simulink model "mainSimulink_localPi"  (R2021a)
settings: Solver=VariableStepAuto  StartTime=0.0  StopTime=inf  FixedStep=samplingTime  RelTol=1e-3
model workspace (MATLAB code in the model file):
  | %% Simulink settings
  | controllerFile = 'directFFcontroller';
  | set_param('mainSimulink_localPi/Subsystem Reference', 'ReferencedSubsystem', controllerFile);
  | %% Display settings
  | scopeTimeSpan = 30;
  | 
  | %% Robot settings (must match Python)
  | sensorFreq = 250;
  | actuatorFreq = 250;
  | PiAddress = '192.168.4.1';
  | PiTCPport = 12345;
  | dataSize = 3;
  | actuatorMin = [0,0,0];                                  %Min relative pressure for actuators [kPa per actuator]
  | actuatorMax = [20,20,20];                                 %Max relative pressure for actuators [kPa per actuator]
  | regulatorMin = -100;                                %Min relative pressure output for regulators [kPa, same for all regulators]
  | regulatorMax = 100;                                 %Max relative pressure output for regulators [kPa, same for all regulators]
  | sensorSamplingTime = 1/sensorFreq;
  | actuatorTime = 1/actuatorFreq;
  | 
  | %% Unity communication settings (must match Unity)
  | UnityAddress = '127.0.0.1';                         %address for Matlab-Unity communication. 127.0.0.1 means local
  | UnityTCPport = 26950;                               %make sure that this port matches the one chosen in Unity
  | nrMessages = 3;                                     %nr of values that you are reading per packet. Depends on your Unity settings
  | UnitysampleFrequency = 120;                         %frequency on Simulink checking TCP connection
  | 
  | %%%ONLY EDIT WHEN THE UNITY MESSAGE TYPE OR HEADER CHANGES%%
  | headerWidth = 12;                                   %nr of bytes in message header (before actual message)
  | signalWidth = 8;                                    %length of each value in message, depends on data type (which is double for now, which is 8 bytes)
  | messageWidth = nrMessages .* signalWidth;           %length of message without header
  | totalMessageWidth = headerWidth + messageWidth;     %length of total packet
  | UnitySamplingTime = 1/UnitysampleFrequency;
undefined symbols (not defined in the file): f
libraries: slrealtimeutilitieslib x4, etargetslib x4, slrealtimeiplib x3, instrumentlib x2
settings Model: EnablePacing=on  Creator=chukh  LastModifiedBy=20210123

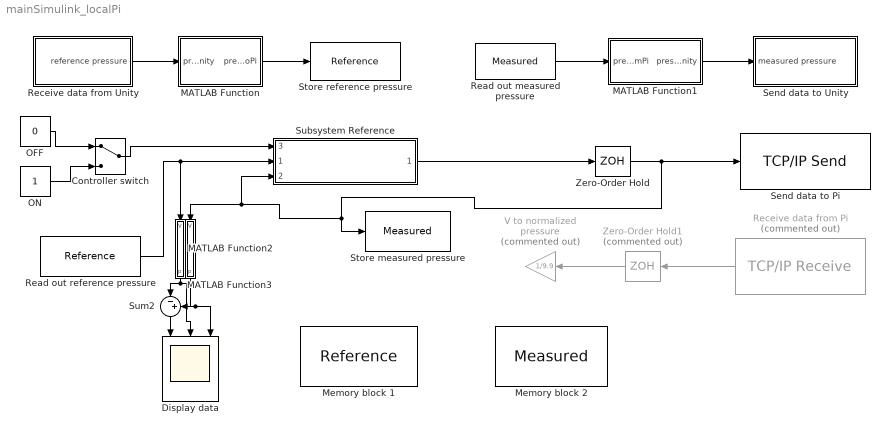
== system mainSimulink_localPi ==
  Controller switch : ManualSwitch
  Display data : Scope  NumInputPorts=3
  MATLAB Function : MATLAB Function  TreatAsAtomicUnit=on
  MATLAB Function1 : MATLAB Function  TreatAsAtomicUnit=on
  MATLAB Function2 : MATLAB Function  TreatAsAtomicUnit=on
  MATLAB Function3 : MATLAB Function  TreatAsAtomicUnit=on
  Memory block 1 : DataStoreMemory  DataStoreName=Reference  ReadBeforeWriteMsg=warning  WriteAfterWriteMsg=warning  WriteAfterReadMsg=warning  InitialValue=zeros(1,dataSize)  ShowAdditionalParam=off  Dimensions=[1 dataSize]
  Memory block 2 : DataStoreMemory  DataStoreName=Measured  ReadBeforeWriteMsg=warning  WriteAfterWriteMsg=warning  WriteAfterReadMsg=warning  InitialValue=zeros(1,dataSize)  ShowAdditionalParam=off  Dimensions=[1 dataSize]
  OFF : Constant  Value=0
  ON : Constant
  Read out measured pressure : DataStoreRead  DataStoreName=Measured  IndexOptions=Index vector (dialog)  Indices=1  OutputSizes=1
  Read out reference pressure : DataStoreRead  DataStoreName=Reference  IndexOptions=Index vector (dialog)  Indices=1  OutputSizes=1
  Receive data from Pi : instrumentlib/TCP//IP Receive  Commented=on  Host=192.168.4.1  Port=PiTCPport  DataSize=dataSize  EnableBlockingMode=on  Timeout=0.5  SampleTime=sensorSamplingTime  DataType=double  ByteOrder=LittleEndian  ASCIIFormatting=%f,  Terminator=LF
  Receive data from Unity : Subsystem
  Send data to Pi : instrumentlib/TCP//IP Send  Host=192.168.4.1  Port=PiTCPport  EnableBlockingMode=on  Timeout=0.5  ByteOrder=LittleEndian  TransferDelay=on
  Send data to Unity : Subsystem
  Store measured pressure : DataStoreWrite  DataStoreName=Measured  IndexOptions=Index vector (dialog)  Indices=1  OutputSizes=1
  Store reference pressure : DataStoreWrite  DataStoreName=Reference  IndexOptions=Index vector (dialog)  Indices=1  OutputSizes=1
  Subsystem Reference : Subsystem  ReferencedSubsystem=directFFcontroller
      settings: PortSchema="{\"entries\":[{\"content\":{\"sides\":[{\"content\":{\"connectorIds\":[\"In3\",\"In1\",\"In2\"]},\"type\":\"ConnectorPlacement.EquallySpacedRectSide\",\"uuid\":\"e7b3a722-e0eb-4523-936c-9c3b79c2c41f\"},{\"content\":{\"connectorIds\":[\"Out1\"],\"side\":\"RIGHT\"},\"type\":\"ConnectorPlacement.EquallySpacedRectSide\",\"uuid\":\"1532b6ae-993f-4a88-9279-fc9a4eded03a\"},{\"content\":{\"connectorIds\":[],\"side\":\"TOP\"},\"type\":\"ConnectorPlacement.EquallySpacedRectSide\",\"uuid\":\"9848284d-3c0a-4259-bac0-7c6aae442a0e\"}]},\"type\":\"ConnectorPlacement.EquallySpacedConnector\",\"uuid\":\"d62a861a-c088-4a48-af1e-4b6a4475476a\"}],\"packageUris\":[\"http://schema.mathworks.com/mf0/Connector/R2020b\"],\"version\":\"1.0\"}"
  Sum2 : Sum  Inputs=|-+
  V to normalized pressure : Gain  Commented=on  Gain=1/9.9
  Zero-Order Hold : ZeroOrderHold  SampleTime=actuatorTime
  Zero-Order Hold1 : ZeroOrderHold  Commented=on  SampleTime=actuatorTime
  wires:
  Zero-Order Hold1/1 -> V to normalized pressure/1
  MATLAB Function2/1(p) -> Sum2/1, Display data/2
  MATLAB Function3/1(p) -> Sum2/2, Display data/3
  Read out reference pressure/1 -> MATLAB Function2/1(V), Subsystem Reference/1
  Sum2/1 -> Display data/1
  Receive data from Unity/1("reference pressure ") -> MATLAB Function/1(pressureFromUnity)
  MATLAB Function/1(pressureToPi) -> Store reference pressure/1
  Read out measured pressure/1 -> MATLAB Function1/1(pressureFromPi)
  Receive data from Pi/1 -> Zero-Order Hold1/1
  Zero-Order Hold/1 -> Subsystem Reference/2, MATLAB Function3/1(V), Store measured pressure/1, Send data to Pi/1
  Subsystem Reference/1 -> Zero-Order Hold/1
  MATLAB Function1/1(pressureToUnity) -> Send data to Unity/1(measured pressure)
  OFF/1 -> Controller switch/1
  ON/1 -> Controller switch/2
  Controller switch/1 -> Subsystem Reference/3

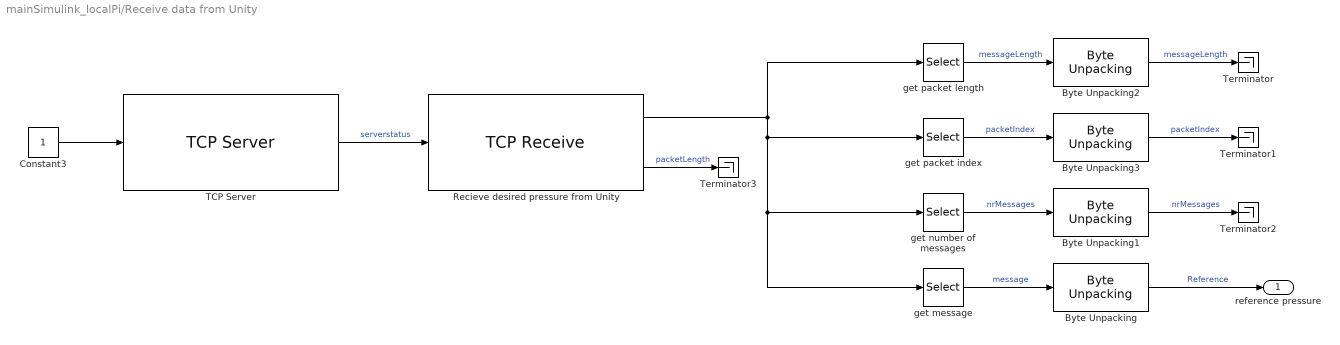
== system mainSimulink_localPi/Receive data from Unity ==
  Byte Unpacking{,1..3} (4 alike) : slrealtimeutilitieslib/Byte Unpacking
      settings: SourceProductBaseCode=XP
  Constant3 : Constant  OutDataTypeStr=double
  Recieve desired pressure from Unity : slrealtimeiplib/TCP Receive  Priority=1  socketAddPortVal=Server: UnityAddress:UnityTCPport  rcvWidth=totalMessageWidth  sampleTime=UnitySamplingTime
      settings: SourceProductBaseCode=XP
  TCP Server : slrealtimeiplib/TCP Server  Priority=-1  useHostTargetConn=off  serverAddress=UnityAddress  serverPort=UnityTCPport
      settings: SourceProductBaseCode=XP
  Terminator{,1..3} (4 alike) : Terminator
  get message : Selector  InputPortWidth=totalMessageWidth  IndexOptions=Index vector (dialog)  Indices=[headerWidth+1:totalMessageWidth]  OutputSizes=1
  get number of messages : Selector  InputPortWidth=totalMessageWidth  IndexOptions=Index vector (dialog)  Indices=[signalWidth+1:headerWidth]  OutputSizes=1
  get packet index : Selector  InputPortWidth=totalMessageWidth  IndexOptions=Index vector (dialog)  Indices=[5:signalWidth]  OutputSizes=1
  get packet length : Selector  InputPortWidth=totalMessageWidth  IndexOptions=Index vector (dialog)  Indices=[1:4]  OutputSizes=1
  "reference pressure " : Outport
  wires:
  TCP Server/1 -> Recieve desired pressure from Unity/1  "serverstatus"
  Recieve desired pressure from Unity/1 -> get packet index/1, get number of messages/1, get message/1, get packet length/1
  Byte Unpacking3/1 -> Terminator1/1  "packetIndex"
  get packet length/1 -> Byte Unpacking2/1  "messageLength"
  get number of messages/1 -> Byte Unpacking1/1  "nrMessages"
  Byte Unpacking1/1 -> Terminator2/1  "nrMessages"
  get packet index/1 -> Byte Unpacking3/1  "packetIndex"
  get message/1 -> Byte Unpacking/1  "message"
  Constant3/1 -> TCP Server/1
  Byte Unpacking2/1 -> Terminator/1  "messageLength"
  Byte Unpacking/1 -> "reference pressure "/1  "Reference"
  Recieve desired pressure from Unity/2 -> Terminator3/1  "packetLength"

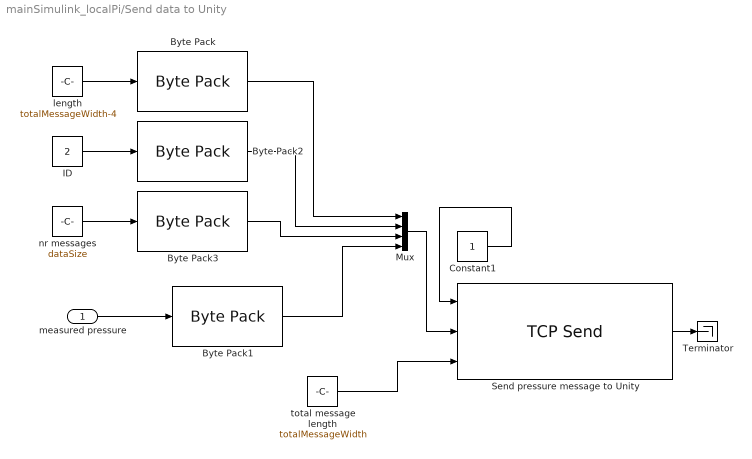
== system mainSimulink_localPi/Send data to Unity ==
  measured pressure : Inport
  Byte Pack : etargetslib/Byte Pack  datatypes={'int32'}  byteAlign=1
  Byte Pack1 : etargetslib/Byte Pack  datatypes={'double'}  byteAlign=1
  Byte Pack2 : etargetslib/Byte Pack  datatypes={'int32'}  byteAlign=1
  Byte Pack3 : etargetslib/Byte Pack  datatypes={'int32'}  byteAlign=1
  Constant1 : Constant
  ID : Constant  Value=2  OutDataTypeStr=int32
  Mux : Mux
  Send pressure message to Unity : slrealtimeiplib/TCP Send  socketAddPortVal=Server: UnityAddress:UnityTCPport  sampleTime=-1
      settings: SourceProductBaseCode=XP
  Terminator : Terminator
  length : Constant  Value=totalMessageWidth-4  OutDataTypeStr=int32
  nr messages : Constant  Value=dataSize  OutDataTypeStr=int32
  total message length : Constant  Value=totalMessageWidth
  wires:
  total message length/1 -> Send pressure message to Unity/3
  Constant1/1 -> Send pressure message to Unity/1
  ID/1 -> Byte Pack2/1
  Byte Pack2/1 -> Mux/2
  length/1 -> Byte Pack/1
  measured pressure/1 -> Byte Pack1/1
  Mux/1 -> Send pressure message to Unity/2
  Byte Pack3/1 -> Mux/3
  Byte Pack1/1 -> Mux/4
  nr messages/1 -> Byte Pack3/1
  Byte Pack/1 -> Mux/1
  Send pressure message to Unity/1 -> Terminator/1

== matlab function mainSimulink_localPi/MATLAB Function ==
  data: pressureFromUnity input size=[1 nrMessages]; regulatorMin parameter size=1; regulatorMax parameter size=1; actuatorMin parameter size=[1 nrMessages]; actuatorMax parameter size=[1 nrMessages]; dataSize parameter size=1; pressureToPi output size=[1 nrMessages]
function pressureToPi = fcn(pressureFromUnity, regulatorMin, regulatorMax, actuatorMin, actuatorMax, dataSize)


zeroToPi = (0 - regulatorMin) ./ (regulatorMax - regulatorMin);
pressureToPi = repmat(zeroToPi,1,dataSize); 

for c=1:dataSize

    if(length(actuatorMin)~=dataSize)
       disp('number of actuators does not match dataSize in Model Workspace'); 
    end
    
    if(pressureFromUnity(c) > 1)
       pressureFromUnity(c) = 1;
       disp('Unity is sending signals > 1');
    end
    
    if(pressureFromUnity(c) < 0)
       pressureFromUnity(c) = 0;
       disp('Unity is sending signals < 0');
    end

minToPi = (actuatorMin(c) - regulatorMin) ./ (regulatorMax - regulatorMin);
maxToPi = (actuatorMax(c) - regulatorMin) ./ (regulatorMax - regulatorMin);   
pressureToPi(c) = minToPi + (maxToPi - minToPi).* pressureFromUnity(c);

end

end

== matlab function mainSimulink_localPi/MATLAB Function2 ==
  data: V input; p output
function p = V2kPa(V)
p = (V-0.5)*200;

== matlab function mainSimulink_localPi/MATLAB Function3 ==
  data: V input; p output
function p = V2kPa(V)
p = (V-0.5)*200;

== matlab function mainSimulink_localPi/MATLAB Function1 ==
  data: pressureFromPi input size=[1 dataSize]; pressureToUnity output size=[1 dataSize]; dataSize parameter size=1; actuatorMin parameter size=[1 dataSize]; actuatorMax parameter size=[1 dataSize]; regulatorMin parameter size=1; regulatorMax parameter size=1
function pressureToUnity = fcn(pressureFromPi,dataSize, actuatorMin, actuatorMax, regulatorMin, regulatorMax)

pressureToUnity = zeros(1,dataSize);                                %initialize with zeros

for c=1:dataSize

minToPi = (actuatorMin(c) - regulatorMin) ./ (regulatorMax - regulatorMin);
maxToPi = (actuatorMax(c) - regulatorMin) ./ (regulatorMax - regulatorMin);
pressureToUnity(c) = (pressureFromPi(c) - minToPi) ./ (maxToPi - minToPi);

end
